simulink library "WECSim_Lib_sp"  (R2014b)
settings: Solver=ode45  StartTime=0.0  StopTime=10.0  RelTol=1e-3
undefined symbols (not defined in the file): body, constraint, pto, simu, waves, X, Y, Z
libraries: nesl_utility x41, sm_lib x36
(part 2 of 2)

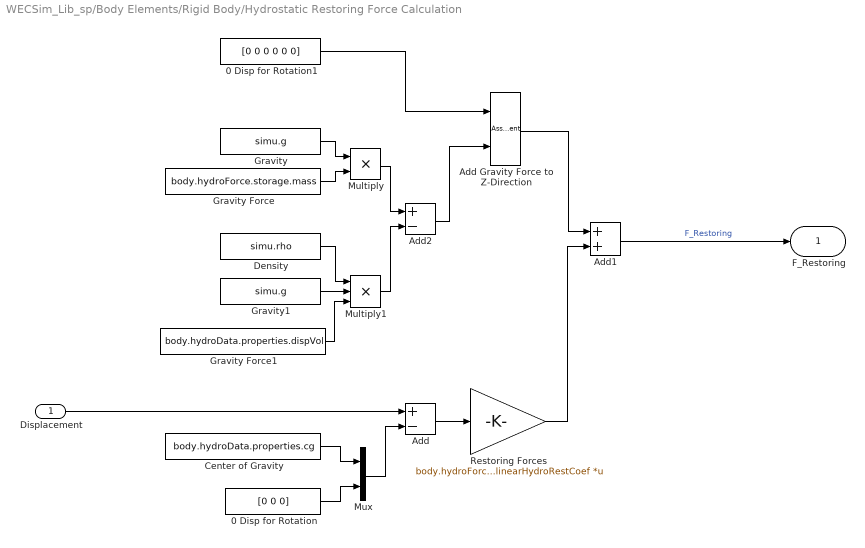
== system WECSim_Lib_sp/Body Elements/Rigid Body/Hydrostatic Restoring Force Calculation ==
  Displacement : Inport
  0 Disp for Rotation : Constant  Value=[0 0 0]
  0 Disp for Rotation1 : Constant  Value=[0 0 0 0 0 0]
  Add : Sum  Inputs=+-
  Add Gravity Force to Z-Direction : Assignment  Indices=3
  Add1 : Sum
  Add2 : Sum  Inputs=+-
  Center of Gravity : Constant  Value=body.hydroData.properties.cg
  Density : Constant  Value=simu.rho
  Gravity : Constant  Value=simu.g
  Gravity Force : Constant  Value=body.hydroForce.storage.mass
  Gravity Force1 : Constant  Value=body.hydroData.properties.dispVol
  Gravity1 : Constant  Value=simu.g
  Multiply : Product  Inputs=**
  Multiply1 : Product  Inputs=***
  Mux : Mux  Inputs=2
  Restoring Forces : Gain  Gain=body.hydroForce.linearHydroRestCoef  Multiplication=Matrix(K*u)
  F_Restoring : Outport
  wires:
  Add/1 -> Restoring Forces/1
  Displacement/1 -> Add/1
  Mux/1 -> Add/2
  Center of Gravity/1 -> Mux/1
  0 Disp for Rotation/1 -> Mux/2
  Gravity/1 -> Multiply/1
  Gravity Force/1 -> Multiply/2
  0 Disp for Rotation1/1 -> Add Gravity Force to Z-Direction/1
  Add Gravity Force to Z-Direction/1 -> Add1/1
  Add1/1 -> F_Restoring/1  "F_Restoring"
  Gravity Force1/1 -> Multiply1/3
  Gravity1/1 -> Multiply1/2
  Density/1 -> Multiply1/1
  Multiply/1 -> Add2/1
  Multiply1/1 -> Add2/2
  Add2/1 -> Add Gravity Force to Z-Direction/2
  Restoring Forces/1 -> Add1/2

== system WECSim_Lib_sp/Body Elements/Rigid Body/Mooring Force Calculation (Map) ==
  Displacement : Inport
  Velocity : Inport  Port=2
  0 Disp for Rotation : Constant  Value=[0 0 0]
  Add : Sum  Inputs=+-
  Center of Gravity : Constant  Value=body.hydroData.properties.cg
  Mooring Damping : Gain  Gain=body.mooring.c  Multiplication=Matrix(K*u)
  Mooring Stiffness : Gain  Gain=body.mooring.k  Multiplication=Matrix(K*u)
  Mooring Pre-Tension : Constant  Value=body.mooring.preTension
  Mux : Mux  Inputs=2
  sum : Sum  Inputs=++-
  F_Mooring : Outport
  wires:
  Mooring Stiffness/1 -> sum/1
  Velocity/1 -> Mooring Damping/1
  Mooring Damping/1 -> sum/2
  sum/1 -> F_Mooring/1  "F_Mooring"
  Mooring Pre-Tension/1 -> sum/3
  Add/1 -> Mooring Stiffness/1
  Mux/1 -> Add/2
  Displacement/1 -> Add/1
  Center of Gravity/1 -> Mux/1
  0 Disp for Rotation/1 -> Mux/2

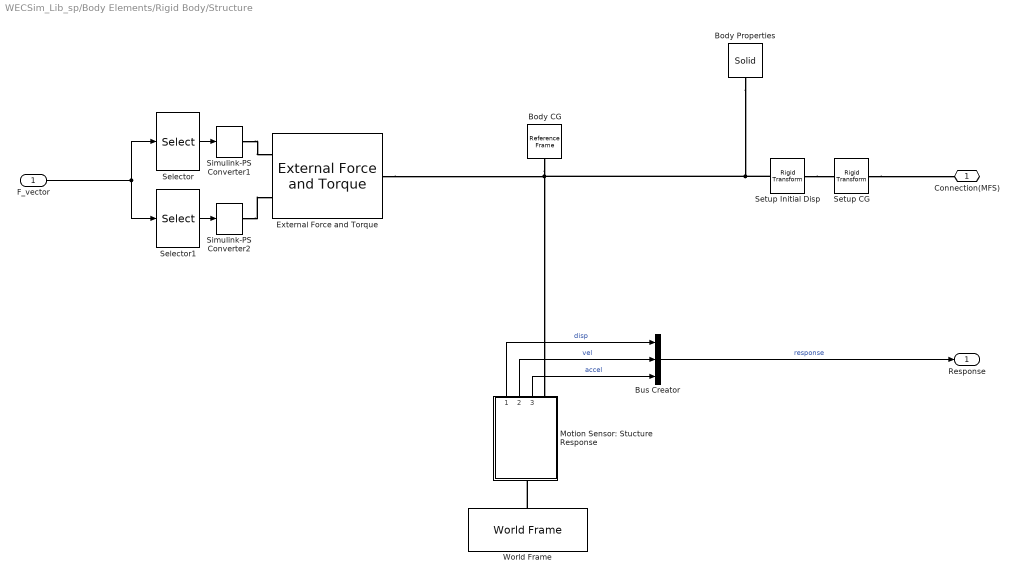
== system WECSim_Lib_sp/Body Elements/Rigid Body/Structure ==
  F_vector : Inport
  Body CG : sm_lib/Frames and Transforms/Reference Frame  BlockFunction=simmechanics.library.frames_transforms.reference_frame
  Body Properties : sm_lib/Body Elements/Solid  InertiaType=Custom  Mass=body.mass  MassUnits=kg  CenterOfMass=[0 0 0]  CenterOfMassUnits=m  MomentsOfInertia=body.momOfInertia  MomentsOfInertiaUnits=kg*m^2  ProductsOfInertia=[0 0 0]  ProductsOfInertiaUnits=kg*m^2  DensityBased=on  Density=1000  DensityUnits=kg/(m^3)  GraphicType=FromGeometry  MarkerShape=Sphere  MarkerSize=10  MarkerSizeUnits=m  GraphicVisPropType=SimpleVisualProperties  GraphicDiffuseColor=[1 1 0]  GraphicSpecularColor=[0.5 0.5 0.5 1.0]  GraphicAmbientColor=[0.15 0.15 0.15 1.0]  GraphicEmissiveColor=[0.0 0.0 0.0 1.0]  GraphicShininess=75  GraphicOpacity=1  GeometryShape=FromFile  RectangleSize=[1 1]  RectangleSizeUnits=m  BrickDimensions=[1 1 1]  BrickDimensionUnits=m  CylinderRadius=1  CylinderRadiusUnits=m  CylinderLength=1  CylinderLengthUnits=m  SphereRadius=1  SphereRadiusUnits=m  EllipsoidRadii=[1 1 1]  EllipsoidRadiiUnits=m  ExtrusionCrossSection=[1 1; -1 1; -1 -1; 1 -1]  ExtrusionCrossSectionUnits=m  ExtrusionLength=1  ExtrusionLengthUnits=m  PolygonNumSides=3  PolygonOuterRadius=1  PolygonOuterRadiusUnits=m  ExtGeomFileType=STL  ExtGeomFileName=geometry/float.stl  ExtGeomFileUnits=m  RevolutionCrossSection=[1 1; 1 -1; 2 -1; 2 1]  RevolutionCrossSectionUnits=m  RevolutionExtent=Full  RevolutionAngle=180  RevolutionAngleUnits=deg  BlockFunction=simmechanics.library.body_elements.solid
  Bus Creator : BusCreator  Inputs=3
  External Force and Torque : sm_lib/Forces and Torques/External Force and Torque  ForceResolutionFrame=World  EnableForceX=off  EnableForceY=off  EnableForceZ=off  EnableForce=on  TorqueResolutionFrame=World  EnableTorqueX=off  EnableTorqueY=off  EnableTorqueZ=off  EnableTorque=on  BlockFunction=simmechanics.library.forces_torques.external_force_torque
  Motion Sensor: Stucture Response : Subsystem
  Selector : Selector  InputPortWidth=6  Indices=[1:3]
  Selector1 : Selector  InputPortWidth=6  Indices=[4:6]
  Setup CG : sm_lib/Frames and Transforms/Rigid Transform  TranslationMethod=Cartesian  TranslationLengthUnit=m  TranslationStandardAxis=+Z  TranslationStandardOffset=0  TranslationCartesianOffset=body.hydroData.properties.cg  TranslationROffset=0  TranslationROffsetUnits=m  TranslationZOffset=0  TranslationZOffsetUnits=m  TranslationThetaOffset=0  TranslationThetaOffsetUnits=deg  RotationMethod=None  RotationAngleUnits=rad  RotationStandardAxis=+Y  RotationAngle=0.05  RotationArbitraryAxis=[0.57735026918962584 0.57735026918962584 0.57735026918962584]  FollAlignAxisA=+X  BaseAlignAxisA=+Y  FollAlignAxisB=+Y  BaseAlignAxisB=+Z  RotationMatrix=[1 0 0; 0 1 0; 0 0 1]  BlockFunction=simmechanics.library.frames_transforms.rigid_transform
  Setup Initial Disp : sm_lib/Frames and Transforms/Rigid Transform  TranslationMethod=Cartesian  TranslationLengthUnit=m  TranslationStandardAxis=+Z  TranslationStandardOffset=0  TranslationCartesianOffset=body.initDisp.initLinDisp  TranslationROffset=0  TranslationROffsetUnits=m  TranslationZOffset=0  TranslationZOffsetUnits=m  TranslationThetaOffset=0  TranslationThetaOffsetUnits=deg  RotationMethod=ArbitraryAxis  RotationAngleUnits=rad  RotationStandardAxis=+Y  RotationAngle=body.initDisp.initAngularDispAngle  RotationArbitraryAxis=body.initDisp.initAngularDispAxis  FollAlignAxisA=+X  BaseAlignAxisA=+Y  FollAlignAxisB=+Y  BaseAlignAxisB=+Z  RotationMatrix=[1 0 0; 0 1 0; 0 0 1]  BlockFunction=simmechanics.library.frames_transforms.rigid_transform
  Simulink-PS Converter1 : nesl_utility/Simulink-PS Converter  PhysicalDomain=network_engine_domain  SubClassName=ps_input  LeftPortType=input  RightPortType=output  PseudoPeriodic=off  Frequencies=[]  NoiseDistribution=none  NoiseParameters=[]  Unit=1  AffineConversion=off  InputFiltering=off  SimscapeFilterOrder=1  InputFilterTimeConstant=0.001  UdotUserProvided=1
  Simulink-PS Converter2 : nesl_utility/Simulink-PS Converter  PhysicalDomain=network_engine_domain  SubClassName=ps_input  LeftPortType=input  RightPortType=output  PseudoPeriodic=off  Frequencies=[]  NoiseDistribution=none  NoiseParameters=[]  Unit=1  AffineConversion=off  InputFiltering=off  SimscapeFilterOrder=1  InputFilterTimeConstant=0.001  UdotUserProvided=1
  World Frame : sm_lib/Frames and Transforms/World Frame  BlockFunction=simmechanics.library.frames_transforms.world_frame
  Connection(MFS) : PMIOPort  Port=1  Side=Right
  Response : Outport
  wires:
  F_vector/1 -> Selector1/1, Selector/1
  Selector/1 -> Simulink-PS Converter1/1
  Selector1/1 -> Simulink-PS Converter2/1
  Bus Creator/1 -> Response/1  "response"
  Motion Sensor: Stucture Response/1(Displacement) -> Bus Creator/1  "disp"
  Motion Sensor: Stucture Response/2(Velocity) -> Bus Creator/2  "vel"
  Motion Sensor: Stucture Response/3(Acceleration) -> Bus Creator/3  "accel"
  connections:
  Simulink-PS Converter1/RConn1 -- External Force and Torque/LConn1
  Simulink-PS Converter2/RConn1 -- External Force and Torque/LConn2
  Setup CG/LConn1 -- Connection(MFS)/RConn1
  Setup Initial Disp/LConn1 -- Setup CG/RConn1
  World Frame/RConn1 -- Motion Sensor: Stucture Response/LConn1
  Setup Initial Disp/RConn1 -- Body Properties/RConn1 -- External Force and Torque/RConn1 -- Body CG/RConn1 -- Motion Sensor: Stucture Response/RConn1

== system WECSim_Lib_sp/Body Elements/Rigid Body/Viscous Damping Force Calculation ==
  Velocity : Inport
  Abs : Abs
  Times : Product  Inputs=**
  Viscous Damping : Gain  Gain=body.hydroForce.visDampingCoef  Multiplication=Matrix(K*u)
  F_Viscous : Outport
  wires:
  Velocity/1 -> Abs/1, Times/1
  Abs/1 -> Times/2
  Times/1 -> Viscous Damping/1
  Viscous Damping/1 -> F_Viscous/1  "F_Viscous"

== system WECSim_Lib_sp/Body Elements/Rigid Body/Wave Diffraction and Excitation Force Calculation ==
  Applied Ramp Function : Subsystem  TreatAsAtomicUnit=on
  If : If  IfExpression=u1 < 20
  If1 : If  NumInputs=2  IfExpression=u1 < u2
  Iregular Wave Excitation Force : Subsystem  TreatAsAtomicUnit=on
  Merge : Merge
  Merge1 : Merge
  No Ramp Function : Subsystem  TreatAsAtomicUnit=on
  Ramp Function Time : Constant  Value=simu.rampT
  Regular Wave Excitation Force : Subsystem  TreatAsAtomicUnit=on
  Wave Type : Constant  Value=waves.typeNum
  F_Excitation : Outport
  wires:
  [Clock] -> Iregular Wave Excitation Force/1(Time), If1/1
  Merge1/1 -> F_Excitation/1  "F_Excitation"
  No Ramp Function/1(Out1) -> Merge1/2
  Applied Ramp Function/1(Out1) -> Merge1/1
  If1/1 -> Applied Ramp Function/Action
  If1/2 -> No Ramp Function/Action
  Merge/1 -> Applied Ramp Function/1(In1), No Ramp Function/1(In1)
  Ramp Function Time/1 -> If1/2
  Iregular Wave Excitation Force/1(F_wave) -> Merge/2
  Regular Wave Excitation Force/1(F_wave) -> Merge/1
  If/2 -> Iregular Wave Excitation Force/Action
  If/1 -> Regular Wave Excitation Force/Action
  Wave Type/1 -> If/1

== system WECSim_Lib_sp/Body Elements/Rigid Body/Wave Radiation Forces Calculation ==
  Velocity : Inport
  Acceleration : Inport  Port=2
  Added Mass Forces : Gain  Gain=body.hydroForce.fAddedMass(1:6,1+(body.bodyNumber-1)*6:6+(body.bodyNumber-1)*6)  Multiplication=Matrix(K*u)
  ConvOption : Constant  Value=simu.convCalc
  Convolution Integral : Subsystem
  Damping Forces : Gain  Gain=body.hydroForce.fDamping(1:6,1+(body.bodyNumber-1)*6:6+(body.bodyNumber-1)*6)  Multiplication=Matrix(K*u)
  If Statement : If
  Merge : Merge
  State-Space-Action : Subsystem  TreatAsAtomicUnit=on
  Sum of Elements : Sum
  Transport Delay : TransportDelay  DelayTime=10e-8
  F_RadiationDamping : Outport
  F_AddedMass : Outport  Port=2
  wires:
  Acceleration/1 -> Transport Delay/1
  Transport Delay/1 -> Added Mass Forces/1
  Sum of Elements/1 -> F_RadiationDamping/1  "F_RadiationDamping"
  Velocity/1 -> State-Space-Action/1(Velin), Convolution Integral/1(Velocity), Damping Forces/1
  Damping Forces/1 -> Sum of Elements/1  "F_Radiation Damping"
  Added Mass Forces/1 -> F_AddedMass/1  "F_AddedMass"
  If Statement/2 -> Convolution Integral/Action
  If Statement/1 -> State-Space-Action/Action
  State-Space-Action/1(Fout) -> Merge/1
  Merge/1 -> Sum of Elements/2  "F_Convolution Integral"
  Convolution Integral/1(F_CI) -> Merge/2
  ConvOption/1 -> If Statement/1

== system WECSim_Lib_sp/PTOs/Rotational PTO (Local RY)/ForceAndPower ==
  Pos : Inport
  Vel : Inport  Port=2
  Add : Sum
  Calculate Power : Product  Inputs=**
  Calculate Power1 : Product  Inputs=**
  Calculate Power2 : Product  Inputs=**
  Math Function : Math  Operator=square  SaturateOnIntegerOverflow=on
  PCC Damping Coefficient : Constant  Value=pto.c
  PCC Stiffness Coefficient : Constant  Value=pto.k
  Force/Torque : Outport
  Power : Outport  Port=2
  wires:
  PCC Damping Coefficient/1 -> Calculate Power/1, Calculate Power1/1
  Calculate Power/1 -> Power/1
  Vel/1 -> Math Function/1, Calculate Power1/2
  PCC Stiffness Coefficient/1 -> Calculate Power2/2
  Pos/1 -> Calculate Power2/1
  Add/1 -> Force/Torque/1
  Math Function/1 -> Calculate Power/2
  Calculate Power2/1 -> Add/1
  Calculate Power1/1 -> Add/2

== system WECSim_Lib_sp/PTOs/Translational PTO (Local X)/ForceAndPower ==
  Pos : Inport
  Vel : Inport  Port=2
  Add : Sum
  Calculate Power : Product  Inputs=**
  Calculate Power1 : Product  Inputs=**
  Calculate Power2 : Product  Inputs=**
  Math Function : Math  Operator=square  SaturateOnIntegerOverflow=on
  PCC Damping Coefficient : Constant  Value=pto.c
  PCC Stiffness Coefficient : Constant  Value=pto.k
  Force : Outport
  Power : Outport  Port=2
  wires:
  PCC Damping Coefficient/1 -> Calculate Power/1, Calculate Power1/1
  Calculate Power/1 -> Power/1
  Vel/1 -> Math Function/1, Calculate Power1/2
  PCC Stiffness Coefficient/1 -> Calculate Power2/2
  Pos/1 -> Calculate Power2/1
  Add/1 -> Force/1
  Math Function/1 -> Calculate Power/2
  Calculate Power2/1 -> Add/1
  Calculate Power1/1 -> Add/2

== system WECSim_Lib_sp/PTOs/Translational PTO (Local Z)/ForceAndPower ==
  Pos : Inport
  Vel : Inport  Port=2
  Add : Sum
  Calculate Power : Product  Inputs=**
  Calculate Power1 : Product  Inputs=**
  Calculate Power2 : Product  Inputs=**
  Math Function : Math  Operator=square  SaturateOnIntegerOverflow=on
  PCC Damping Coefficient : Constant  Value=pto.c
  PCC Stiffness Coefficient : Constant  Value=pto.k
  Force : Outport
  Power : Outport  Port=2
  wires:
  PCC Damping Coefficient/1 -> Calculate Power/1, Calculate Power1/1
  Calculate Power/1 -> Power/1
  Vel/1 -> Math Function/1, Calculate Power1/2
  PCC Stiffness Coefficient/1 -> Calculate Power2/2
  Pos/1 -> Calculate Power2/1
  Add/1 -> Force/1
  Math Function/1 -> Calculate Power/2
  Calculate Power2/1 -> Add/1
  Calculate Power1/1 -> Add/2

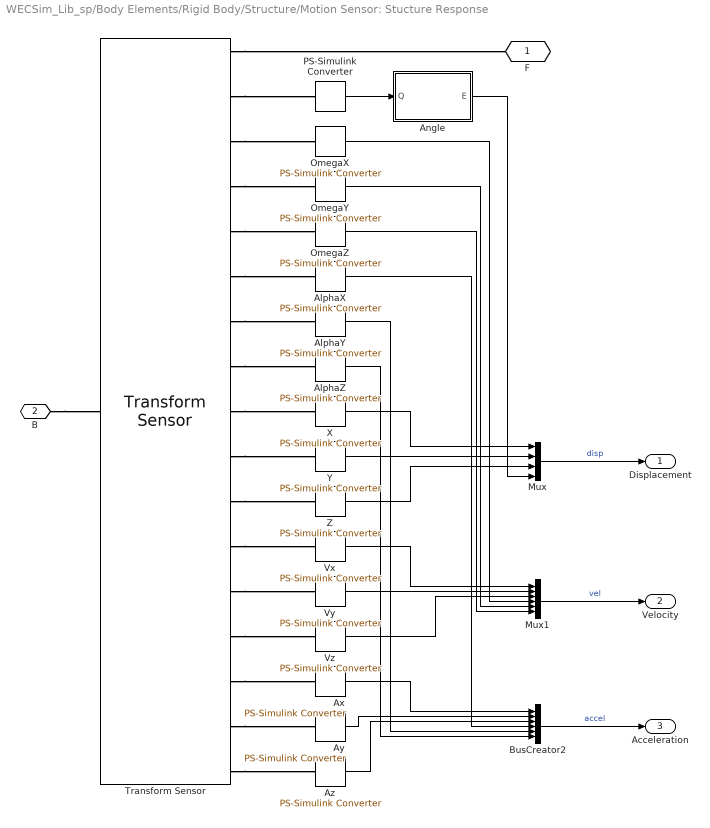
== system WECSim_Lib_sp/Body Elements/Rigid Body/Structure/Motion Sensor: Stucture Response ==
  AlphaX : nesl_utility/PS-Simulink Converter  PhysicalDomain=network_engine_domain  SubClassName=ps_output  LeftPortType=input  RightPortType=output  PseudoPeriodic=off  Frequencies=[]  Unit=1  AffineConversion=off
  "AlphaY " : nesl_utility/PS-Simulink Converter  PhysicalDomain=network_engine_domain  SubClassName=ps_output  LeftPortType=input  RightPortType=output  PseudoPeriodic=off  Frequencies=[]  Unit=1  AffineConversion=off
  AlphaZ : nesl_utility/PS-Simulink Converter  PhysicalDomain=network_engine_domain  SubClassName=ps_output  LeftPortType=input  RightPortType=output  PseudoPeriodic=off  Frequencies=[]  Unit=1  AffineConversion=off
  Angle : MATLAB Function  TreatAsAtomicUnit=on
  Ax : nesl_utility/PS-Simulink Converter  PhysicalDomain=network_engine_domain  SubClassName=ps_output  LeftPortType=input  RightPortType=output  PseudoPeriodic=off  Frequencies=[]  Unit=1  AffineConversion=off
  Ay : nesl_utility/PS-Simulink Converter  PhysicalDomain=network_engine_domain  SubClassName=ps_output  LeftPortType=input  RightPortType=output  PseudoPeriodic=off  Frequencies=[]  Unit=1  AffineConversion=off
  Az : nesl_utility/PS-Simulink Converter  PhysicalDomain=network_engine_domain  SubClassName=ps_output  LeftPortType=input  RightPortType=output  PseudoPeriodic=off  Frequencies=[]  Unit=1  AffineConversion=off
  BusCreator2 : BusCreator  Inputs=6
  Mux : Mux
  Mux1 : Mux  Inputs=6
  OmegaX : nesl_utility/PS-Simulink Converter  PhysicalDomain=network_engine_domain  SubClassName=ps_output  LeftPortType=input  RightPortType=output  PseudoPeriodic=off  Frequencies=[]  Unit=1  AffineConversion=off
  OmegaY : nesl_utility/PS-Simulink Converter  PhysicalDomain=network_engine_domain  SubClassName=ps_output  LeftPortType=input  RightPortType=output  PseudoPeriodic=off  Frequencies=[]  Unit=1  AffineConversion=off
  OmegaZ : nesl_utility/PS-Simulink Converter  PhysicalDomain=network_engine_domain  SubClassName=ps_output  LeftPortType=input  RightPortType=output  PseudoPeriodic=off  Frequencies=[]  Unit=1  AffineConversion=off
  PS-Simulink Converter : nesl_utility/PS-Simulink Converter  PhysicalDomain=network_engine_domain  SubClassName=ps_output  LeftPortType=input  RightPortType=output  PseudoPeriodic=off  Frequencies=[]  Unit=1  AffineConversion=off
  Transform Sensor : sm_lib/Frames and Transforms/Transform Sensor  MeasurementFrame=World  SenseAngle=off  SenseAxis=off  SenseAngle1=off  SenseAngle2=off  SenseAngle3=off  SenseQ=on  SenseR=off  SenseOmegaX=on  SenseOmegaY=on  SenseOmegaZ=on  SenseOmega1=off  SenseOmega2=off  SenseOmega3=off  SenseQDot=off  SenseRDot=off  SenseAlphaX=on  SenseAlphaY=on  SenseAlphaZ=on  SenseAlpha1=off  SenseAlpha2=off  SenseAlpha3=off  SenseQDDot=off  SenseRDDot=off  SenseX=on  SenseY=on  SenseZ=on  SenseRad=off  SenseAzim=off  SenseDist=off  SenseInc=off  SenseXDot=on  SenseYDot=on  SenseZDot=on  SenseRadDot=off  SenseAzimDot=off  SenseDistDot=off  SenseIncDot=off  SenseXDDot=on  SenseYDDot=on  SenseZDDot=on  SenseRadDDot=off  SenseAzimDDot=off  SenseDistDDot=off  SenseIncDDot=off  BlockFunction=simmechanics.library.frames_transforms.transform_sensor
  Vx : nesl_utility/PS-Simulink Converter  PhysicalDomain=network_engine_domain  SubClassName=ps_output  LeftPortType=input  RightPortType=output  PseudoPeriodic=off  Frequencies=[]  Unit=1  AffineConversion=off
  Vy : nesl_utility/PS-Simulink Converter  PhysicalDomain=network_engine_domain  SubClassName=ps_output  LeftPortType=input  RightPortType=output  PseudoPeriodic=off  Frequencies=[]  Unit=1  AffineConversion=off
  Vz : nesl_utility/PS-Simulink Converter  PhysicalDomain=network_engine_domain  SubClassName=ps_output  LeftPortType=input  RightPortType=output  PseudoPeriodic=off  Frequencies=[]  Unit=1  AffineConversion=off
  X : nesl_utility/PS-Simulink Converter  PhysicalDomain=network_engine_domain  SubClassName=ps_output  LeftPortType=input  RightPortType=output  PseudoPeriodic=off  Frequencies=[]  Unit=1  AffineConversion=off
  Y : nesl_utility/PS-Simulink Converter  PhysicalDomain=network_engine_domain  SubClassName=ps_output  LeftPortType=input  RightPortType=output  PseudoPeriodic=off  Frequencies=[]  Unit=1  AffineConversion=off
  Z : nesl_utility/PS-Simulink Converter  PhysicalDomain=network_engine_domain  SubClassName=ps_output  LeftPortType=input  RightPortType=output  PseudoPeriodic=off  Frequencies=[]  Unit=1  AffineConversion=off
  F : PMIOPort  Port=1  Side=Right
  B : PMIOPort  Port=2  Side=Left
  Displacement : Outport
  Velocity : Outport  Port=2
  Acceleration : Outport  Port=3
  wires:
  PS-Simulink Converter/1 -> Angle/1(Q)
  AlphaX/1 -> BusCreator2/4
  Vx/1 -> Mux1/1
  Vy/1 -> Mux1/2
  Vz/1 -> Mux1/3
  Ax/1 -> BusCreator2/1
  Ay/1 -> BusCreator2/2
  Az/1 -> BusCreator2/3
  Mux/1 -> Displacement/1  "disp"
  Mux1/1 -> Velocity/1  "vel"
  BusCreator2/1 -> Acceleration/1  "accel"
  Angle/1(E) -> Mux/4
  X/1 -> Mux/1
  Y/1 -> Mux/2
  Z/1 -> Mux/3
  "AlphaY "/1 -> BusCreator2/5
  AlphaZ/1 -> BusCreator2/6
  OmegaX/1 -> Mux1/4
  OmegaY/1 -> Mux1/5
  OmegaZ/1 -> Mux1/6
  connections:
  Transform Sensor/RConn1 -- F/RConn1
  B/RConn1 -- Transform Sensor/LConn1
  Transform Sensor/RConn2 -- PS-Simulink Converter/LConn1
  Transform Sensor/RConn17 -- Az/LConn1
  Transform Sensor/RConn16 -- Ay/LConn1
  Transform Sensor/RConn15 -- Ax/LConn1
  Transform Sensor/RConn14 -- Vz/LConn1
  Transform Sensor/RConn13 -- Vy/LConn1
  Transform Sensor/RConn12 -- Vx/LConn1
  Transform Sensor/RConn11 -- Z/LConn1
  Transform Sensor/RConn10 -- Y/LConn1
  Transform Sensor/RConn9 -- X/LConn1
  Transform Sensor/RConn6 -- AlphaX/LConn1
  Transform Sensor/RConn7 -- "AlphaY "/LConn1
  Transform Sensor/RConn8 -- AlphaZ/LConn1
  Transform Sensor/RConn3 -- OmegaX/LConn1
  Transform Sensor/RConn4 -- OmegaY/LConn1
  Transform Sensor/RConn5 -- OmegaZ/LConn1

== system WECSim_Lib_sp/Body Elements/Rigid Body/Wave Diffraction and Excitation Force Calculation/Applied Ramp Function ==
  In1 : Inport
  Action Port : ActionPort  ActionType=then
  Add : Sum
  Constant : Constant  Value=2
  Constant1 : Constant
  Divide : Product  Inputs=**/
  Sine Wave : Sin  Frequency=pi/simu.rampT  Phase=pi+pi/2  SampleTime=0
  Out1 : Outport
  wires:
  Add/1 -> Divide/2
  Sine Wave/1 -> Add/2
  Constant1/1 -> Add/1
  Constant/1 -> Divide/3
  Divide/1 -> Out1/1
  In1/1 -> Divide/1

== system WECSim_Lib_sp/Body Elements/Rigid Body/Wave Diffraction and Excitation Force Calculation/Iregular Wave Excitation Force ==
  Time : Inport
  Action Port : ActionPort  ActionType=else
  Excitation Re Part2 : Constant  Value=body.hydroForce.fExt.re  VectorParams1D=off
  Excitation Re Part3 : Constant  Value=body.hydroForce.fExt.im  VectorParams1D=off
  For Each Subsystem : Subsystem  TreatAsAtomicUnit=on
  Sum of Elements : Sum  Inputs=+  CollapseMode=Specified dimension
  dw1 : Constant  Value=(waves.w(end)-waves.w(1))/(waves.numFreq-1)  VectorParams1D=off
  wave frequency : Constant  Value=waves.w  VectorParams1D=off
  wave frequency1 : Constant  Value=waves.phaseRand'  VectorParams1D=off
  wave spectrum : Constant  Value=waves.A*2  VectorParams1D=off
  F_wave : Outport  PortDimensions=6
  wires:
  dw1/1 -> For Each Subsystem/6(dw)
  wave frequency1/1 -> For Each Subsystem/7(phaseRand)
  Sum of Elements/1 -> F_wave/1
  Time/1 -> For Each Subsystem/5(Time)
  For Each Subsystem/1(Out1) -> Sum of Elements/1
  wave spectrum/1 -> For Each Subsystem/1(wave amplitude)
  wave frequency/1 -> For Each Subsystem/2(wave freq)
  Excitation Re Part3/1 -> For Each Subsystem/4(wave fExt im)
  Excitation Re Part2/1 -> For Each Subsystem/3(wave fExt re)

== system WECSim_Lib_sp/Body Elements/Rigid Body/Wave Diffraction and Excitation Force Calculation/No Ramp Function ==
  In1 : Inport
  Action Port : ActionPort  ActionType=else
  Out1 : Outport
  wires:
  In1/1 -> Out1/1

== system WECSim_Lib_sp/Body Elements/Rigid Body/Wave Diffraction and Excitation Force Calculation/Regular Wave Excitation Force ==
  Action Port : ActionPort  ActionType=then
  Add : Sum  Inputs=+-
  BEM Excitation Im Part1 : Constant  Value=body.hydroForce.fExt.im(1,:)  VectorParams1D=off
  BEM Excitation Re Part : Constant  Value=body.hydroForce.fExt.re(1,:)  VectorParams1D=off
  Cos Wave : Sin  Amplitude=waves.A(1,:)  Frequency=waves.w(1,:)  Phase=pi/2  SampleTime=0
  Product : Product  Inputs=**
  Product1 : Product  Inputs=**
  Sin Wave : Sin  Amplitude=waves.A(1,:)  Frequency=waves.w(1,:)  SampleTime=0
  F_wave : Outport  PortDimensions=6
  wires:
  Add/1 -> F_wave/1
  Product/1 -> Add/1
  BEM Excitation Im Part1/1 -> Product1/2
  Product1/1 -> Add/2
  Sin Wave/1 -> Product1/1
  BEM Excitation Re Part/1 -> Product/2
  Cos Wave/1 -> Product/1

== system WECSim_Lib_sp/Body Elements/Rigid Body/Wave Radiation Forces Calculation/Convolution Integral ==
  Velocity : Inport
  Action Port : ActionPort  ActionType=else
  Fluid Memory : MATLAB Function  TreatAsAtomicUnit=on
  Impulse Response Function K : Constant  Value=body.hydroForce.irkb(:,1:6,1+(body.bodyNumber-1)*6:6+(body.bodyNumber-1)*6)
  Time (relative to the current time step) : Constant  Value=simu.CTTime
  Wave Type : Constant  Value=waves.typeNum
  F_CI : Outport
  wires:
  Velocity/1 -> Fluid Memory/2(v)
  Fluid Memory/1(F_FM) -> F_CI/1  "F_Convolution Integral"
  Wave Type/1 -> Fluid Memory/1(check)
  Impulse Response Function K/1 -> Fluid Memory/3(IRKB)
  Time (relative to the current time step)/1 -> Fluid Memory/4(CTTime)

== system WECSim_Lib_sp/Body Elements/Rigid Body/Wave Radiation Forces Calculation/State-Space-Action ==
  Velin : Inport
  Action Port : ActionPort
  State-Space : StateSpace  A=body.hydroForce.ssRadf.A  B=body.hydroForce.ssRadf.B  C=body.hydroForce.ssRadf.C  D=body.hydroForce.ssRadf.D  X0=0
  Fout : Outport
  wires:
  State-Space/1 -> Fout/1
  Velin/1 -> State-Space/1

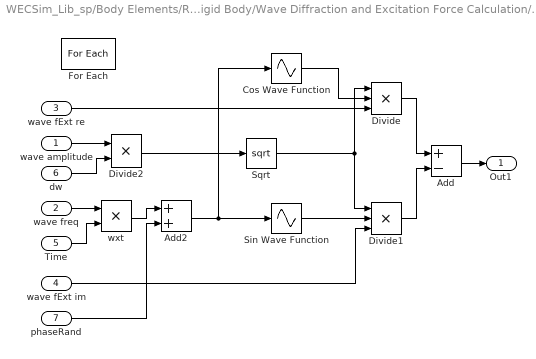
== system WECSim_Lib_sp/Body Elements/Rigid Body/Wave Diffraction and Excitation Force Calculation/Iregular Wave Excitation Force/For Each Subsystem ==
  wave amplitude : Inport  Partition=on  PartitionDimension=1  PartitionWidth=1
  wave freq : Inport  Port=2  Partition=on  PartitionDimension=1  PartitionWidth=1
  wave fExt re : Inport  Port=3  Partition=on  PartitionDimension=1  PartitionWidth=1
  wave fExt im : Inport  Port=4  Partition=on  PartitionDimension=1  PartitionWidth=1
  Time : Inport  Port=5  Partition=off
  dw : Inport  Port=6  Partition=off
  phaseRand : Inport  Port=7  Partition=on  PartitionDimension=1  PartitionWidth=1
  Add : Sum  Inputs=+-
  Add2 : Sum
  Cos Wave Function : Sin  TimeSource=Use external signal  Phase=pi/2  SampleTime=0
  Divide : Product  Inputs=***
  Divide1 : Product  Inputs=***
  Divide2 : Product  Inputs=**
  For Each : ForEach  DisableCoverage=on  IndexMode=One-based
  Sin Wave Function : Sin  TimeSource=Use external signal  SampleTime=0
  Sqrt : Sqrt  SaturateOnIntegerOverflow=on
  wxt : Product  Inputs=**
  Out1 : Outport  ConcatenationDimension=1
  wires:
  Add2/1 -> Cos Wave Function/1, Sin Wave Function/1
  phaseRand/1 -> Add2/2
  wxt/1 -> Add2/1
  Sqrt/1 -> Divide/1, Divide1/1
  Divide2/1 -> Sqrt/1
  dw/1 -> Divide2/2
  wave amplitude/1 -> Divide2/1
  Time/1 -> wxt/2
  Add/1 -> Out1/1
  Cos Wave Function/1 -> Divide/2
  wave fExt re/1 -> Divide/3
  wave freq/1 -> wxt/1
  Sin Wave Function/1 -> Divide1/2
  wave fExt im/1 -> Divide1/3
  Divide/1 -> Add/1
  Divide1/1 -> Add/2

== matlab function WECSim_Lib_sp/Body Elements/Rigid Body/Wave Radiation Forces Calculation/Convolution Integral/Fluid Memory ==
  data: check input; v input; F_FM output; IRKB input; CTTime input
function F_FM = ConvolutionalIntegral(check,v,IRKB,CTTime)

%define persistent variables
persistent velocity;
persistent kkk
len = length(CTTime);

if check==10
    tmpT = zeros(6,1);
else
    if isempty(velocity)
       velocity = zeros(6,len);
       kkk=0;
    else
       kkk=kkk+1;         
       int2=abs(kkk-floor(kkk/5)*5-1);
       if int2<0.00000001
          velocity(:,2:end) = velocity(:,1:end-1);
       end
       velocity(:,1) = v(:);
    end 
    
	%integrate
    tmpT = zeros(6,1);
    for kd=1:6
        tmpV = zeros(len,1);
        for kk=1:6
            tmpY=IRKB(:,kd,kk).*velocity(kk,:)';
            tmpV = tmpV + tmpY;
        end
        tmpT(kd) = trapz(CTTime,tmpV);
    end
end
F_FM=tmpT;
end

== matlab function WECSim_Lib_sp/Body Elements/Rigid Body/Structure/Motion Sensor: Stucture Response/Angle ==
  data: Q input; E output
function E  = EulerAngle(Q)
%#codegen
E=zeros(3,1);
E(1) = atan2( (2*(Q(1)*Q(2)+Q(3)*Q(4))), (1-2* (Q(2)^2+Q(3)^2) ) );
E(2) = asin( 2* (Q(1)*Q(3) - Q(4)*Q(2)));
E(3) = atan2( (2*(Q(1)*Q(4)+Q(2)*Q(3))), (1-2* (Q(3)^2+Q(4)^2) ) );
